simulink model "MPCtesting"  (R2023a)
settings: Solver=ode4  StartTime=0.0  StopTime=4800  FixedStep=0.1  RelTol=1e-3
libraries: slpidlib x1
settings Model: Creator=toma  LastModifiedBy=toma

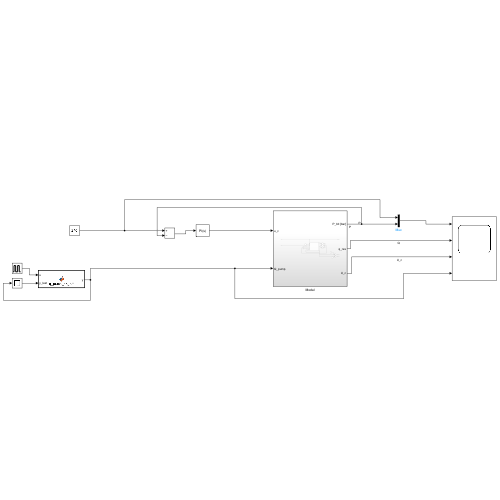
[thumbnail: Simulink's stored preview of the top-level diagram]
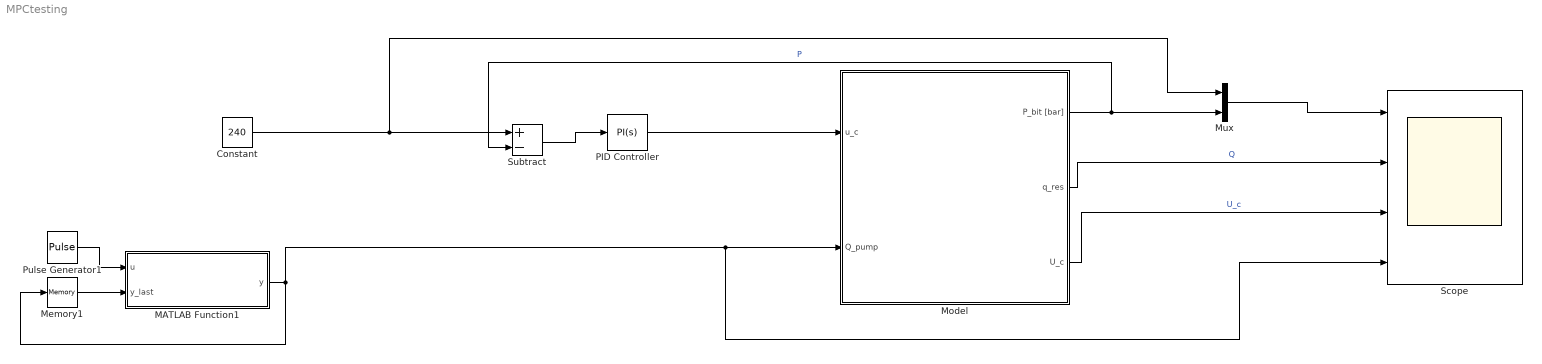
== system MPCtesting ==
  Constant : Constant  Value=240
  MATLAB Function1 : MATLAB Function  TreatAsAtomicUnit=on
  Memory1 : Memory
  Model : Subsystem
  Mux : Mux  Inputs=2
  PID Controller : slpidlib/PID Controller  Controller=PI  Form=Ideal  TimeDomain=Continuous-time  UseExternalTs=off  SampleTime=-1  IntegratorMethod=Forward Euler  FilterMethod=Forward Euler  ControllerParametersSource=internal  P=1  I=1000000000  UseKiTs=off  D=0  N=100  UseFilter=on  TunerSelectOption=Transfer Function Based (PID Tuner App)  InitialConditionSource=internal  InitialConditionForIntegrator=0  InitialConditionForFilter=0  DifferentiatorICPrevScaledInput=0  ExternalReset=none  TrackingMode=off  Kt=1  LimitOutput=off  SatLimitsSource=internal  UpperSaturationLimit=inf  LowerSaturationLimit=-inf  LinearizeAsGain=on  AntiWindupMode=none  Kb=1  LimitIntegrator=off  UpperIntegratorSaturationLimit=inf  LowerIntegratorSaturationLimit=-inf  POutMin=[]  POutMax=[]  IOutMin=[]  IOutMax=[]  DOutMin=[]  DOutMax=[]  NOutMin=[]  NOutMax=[]  SumOutMin=[]  SumOutMax=[]  SaturationOutMin=[]  SaturationOutMax=[]  PParamMin=[]  PParamMax=[]  IParamMin=[]  IParamMax=[]  DParamMin=[]  DParamMax=[]  NParamMin=[]  NParamMax=[]  KbParamMin=[]  KbParamMax=[]  KtParamMin=[]  KtParamMax=[]  KbOutMin=[]  KbOutMax=[]  KtOutMin=[]  KtOutMax=[]  IntegratorOutMin=[]  IntegratorOutMax=[]  FilterOutMin=[]  FilterOutMax=[]  SumI1OutMin=[]  SumI1OutMax=[]  SumI2OutMin=[]  SumI2OutMax=[]  SumI3OutMin=[]  SumI3OutMax=[]  SumI4OutMin=[]  SumI4OutMax=[]  SumDOutMin=[]  SumDOutMax=[]  DifferentiatorOutMin=[]  DifferentiatorOutMax=[]  FilterDiffOutCoefMin=[]  FilterDiffOutCoefMax=[]  ReciprocalOutMin=[]  ReciprocalOutMax=[]  SumDenOutMin=[]  SumDenOutMax=[]  SumNumOutMin=[]  SumNumOutMax=[]  DivideOutMin=[]  DivideOutMax=[]  UdiffTsProdOutMin=[]  UdiffTsProdOutMax=[]  NTsProdOutMin=[]  NTsProdOutMax=[]  UintegralTsProdOutMin=[]  UintegralTsProdOutMax=[]  UngainTsProdOutMin=[]  UngainTsProdOutMax=[]  ClampingZeroOutDataTypeStr=Inherit: Inherit via back propagation  ClampingZeroOutMin=[]  ClampingZeroOutMax=[]  FilterDenConstantOutDataTypeStr=Inherit: Inherit via back propagation  FilterDenConstantOutMin=[]  FilterDenConstantOutMax=[]  PCopyOutDataTypeStr=Inherit: Inherit via back propagation  PCopyOutMin=[]  PCopyOutMax=[]  NCopyOutDataTypeStr=Inherit: Inherit via back propagation  NCopyOutMin=[]  NCopyOutMax=[]  IntegratorContinuousStateAttributes=''  IntegratorStateMustResolveToSignalObject=off  IntegratorRTWStateStorageClass=Auto  FilterContinuousStateAttributes=''  FilterStateMustResolveToSignalObject=off  FilterRTWStateStorageClass=Auto  ParallelPVariant=Passthrough  IdealPVariant=InternalParameters  IVariant=InternalParameters  DVariant=Disabled  IntegratorVariant=Continuous  SatVariant=Disabled  AWVariant=Passthrough  PCopyVariant=Disabled  TRVariant=Disabled  FdbkBlocksVariant=Forward  IdealPFdbkVariant=Disabled  SatFdbkVariant=Disabled  DerivativeFilterVariant=Disabled  NVariant=Disabled  NCopyVariant=Disabled_SignalSpec  FilterICVariant=Disabled  IntegratorICVariant=InternalICs  ExternalResetVariant=Disabled  TRSumVariant=Passthrough  SumFdbkVariant=Disabled  SumVariant=Sum_PI  TsampFilterVariant=InternalTs  TsampNgainVariant=Passthrough  TsampIntegralVariant=Disabled_SignalSpec  ExternalSaturationOutDataTypeStr=Inherit: Same as second input
  Pulse Generator1 : DiscretePulseGenerator  PulseType=Time based  Amplitude=0.025  Period=4500  PulseWidth=50
  Scope : Scope  NumInputPorts=4
  Subtract : Sum  Inputs=+-
  wires:
  Subtract/1 -> PID Controller/1
  Constant/1 -> Mux/1, Subtract/1
  Pulse Generator1/1 -> MATLAB Function1/1(u)
  MATLAB Function1/1(y) -> Memory1/1, Scope/4, Model/2(Q_pump)
  Memory1/1 -> MATLAB Function1/2(y_last)
  Model/2(q_res) -> Scope/2  "Q"
  Model/3(U_c) -> Scope/3  "U_c"
  Model/1(P_bit [bar]) -> Subtract/2, Mux/2  "P"
  Mux/1 -> Scope/1
  PID Controller/1 -> Model/1(u_c)

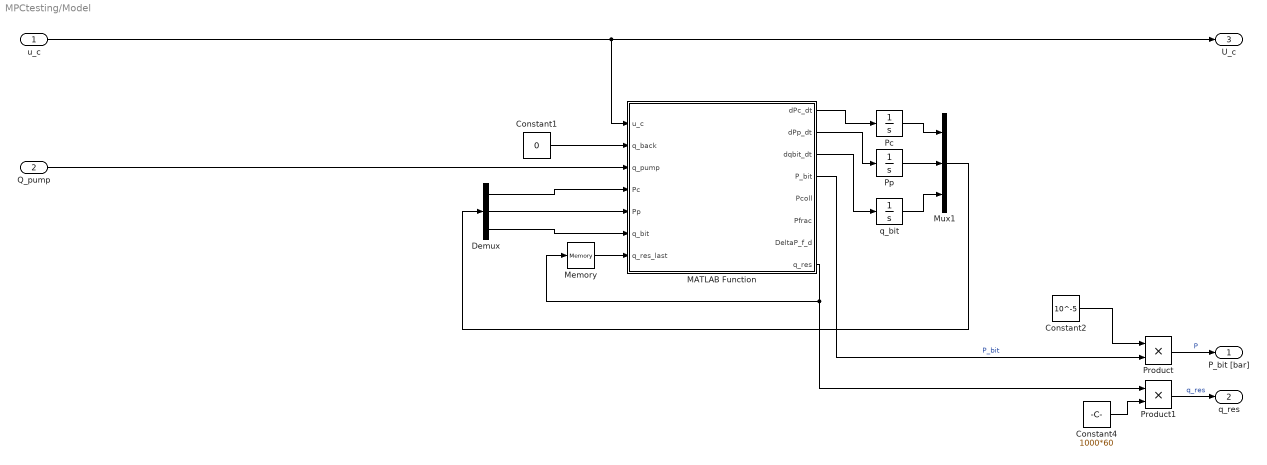
== system MPCtesting/Model ==
  u_c : Inport
  Q_pump : Inport  Port=2
  Constant1 : Constant  Value=0
  Constant2 : Constant  Value=10^-5
  Constant4 : Constant  Value=1000*60
  Demux : Demux  Outputs=3
  MATLAB Function : MATLAB Function  TreatAsAtomicUnit=on
  Memory : Memory
  Mux1 : Mux  Inputs=3
  Pc : Integrator  InitialCondition=4*10^5
  Pp : Integrator  InitialCondition=4*10^5
  Product : Product
  Product1 : Product
  q_bit : Integrator  InitialCondition=0.025
  P_bit [bar] : Outport
  q_res : Outport  Port=2
  U_c : Outport  Port=3
  wires:
  Constant1/1 -> MATLAB Function/2(q_back)
  Mux1/1 -> Demux/1
  q_bit/1 -> Mux1/3
  MATLAB Function/8(q_res) -> Product1/1, Memory/1
  Demux/2 -> MATLAB Function/5(Pp)
  Demux/1 -> MATLAB Function/4(Pc)
  Demux/3 -> MATLAB Function/6(q_bit)
  Pp/1 -> Mux1/2
  Q_pump/1 -> MATLAB Function/3(q_pump)
  Pc/1 -> Mux1/1
  Memory/1 -> MATLAB Function/7(q_res_last)
  MATLAB Function/2(dPp_dt) -> Pp/1
  MATLAB Function/1(dPc_dt) -> Pc/1
  u_c/1 -> U_c/1, MATLAB Function/1(u_c)
  MATLAB Function/3(dqbit_dt) -> q_bit/1
  Product/1 -> P_bit [bar]/1  "P"
  Constant2/1 -> Product/1
  MATLAB Function/4(P_bit) -> Product/2  "P_bit"
  Constant4/1 -> Product1/2
  Product1/1 -> q_res/1  "q_res"

== matlab function MPCtesting/MATLAB Function1 ==
  data: u input; y output; y_last input
function y = q_pump_on_off(u, y_last)

maximum = 0.025;

if y_last < u
    y = y_last + ((1*maximum)/1000);
elseif y_last > u
    y = y_last - (1*maximum/1000);
else 
    y = u;
end

y_last = y;

== matlab function MPCtesting/Model/MATLAB Function ==
  data: dPc_dt output; u_c input; q_back input; q_pump input; Pc input; Pp input; q_bit input; dPp_dt output; dqbit_dt output; P_bit output; Pcoll output; Pfrac output; DeltaP_f_d output; q_res_last input; q_res output
function [dPc_dt, dPp_dt, dqbit_dt, P_bit, Pcoll, Pfrac, DeltaP_f_d, q_res] = OilWell(u_c, q_back, q_pump, Pc, Pp, q_bit, q_res_last)

%Density
rho_l = 1150;
rho_water = 1000;

%Others
WC = 0.1;
PI = 1.6667*10^-9;
Betta_d = 3*10^8;
Betta_a = 2.4*10^8;
g = 9.81;
f_d = 0.02;

%Area
Ad = 0.0067;
Aa = 0.278;

%Hight
Dd = 0.0925;
Da = 0.211;
L = 1600;

%Pressure
Pres = 250*10^5;
Pfrac = 270*10^5;
Pcoll = 220*10^5;
Pbit_ref = 215*10^5;
P0 = 4*10^5;

%Equations:
rho_mix = rho_water*WC + (1-WC)*rho_l;

%v = q_bit/Aa;

DeltaP_f_a = (f_d*L*rho_mix*((q_bit+q_res_last)/Aa)^2)/(2*Da);
DeltaP_f_d = (f_d*L*rho_l*(q_pump/Ad)^2)/(2*Dd);


P_bit = Pc + rho_mix*g*L + DeltaP_f_a;



q_res = max(PI*(Pres-P_bit),0);

N6 = 27.3/(3600*sqrt(10^5));

if u_c < 5  
    Z_c = 0;
elseif u_c >= 5 && u_c < 50
    Z_c = 0.111*u_c-0.557;
else
    Z_c = 0.5*u_c-20;
end

q_choke = N6*Z_c*sqrt(max((Pc-P0),0)/rho_mix);

%differential equatios
dPp_dt = Betta_d/(Ad*L) * (q_pump - q_bit); 

dqbit_dt = (Ad/(rho_l*L) * (Pp + rho_l*g*L - DeltaP_f_d - P_bit));

if q_bit <= 0 && dqbit_dt < 0
    q_bit = 0;
    dqbit_dt = 0;
end

dPc_dt = Betta_a/(Aa*L) * (q_bit + q_res + q_back - q_choke);
